simulink model "Quadcopter"  (R2023b)
settings: Solver=VariableStepAuto  StartTime=0.0  StopTime=10  FixedStep=0.002  RelTol=1e-3  EnableMultiTasking=on
libraries: matrix_library x4, shared6dof x1, robotcorelib x1, uavutilslib x1
settings Model: ExtModeTrigDuration=10000  Creator=plad  LastModifiedBy=plad
settings SolverCC: AlgebraicLoopSolver=TrustRegion  PositivePriorityOrder=on
settings DataIOCC: ReturnWorkspaceOutputs=off
settings OptimizationCC: LifeSpan=inf
settings DebuggingCC: UnconnectedInputMsg=warning  UnconnectedOutputMsg=warning  UnconnectedLineMsg=warning  ArithmeticOperatorsInVariantConditions=warning
settings ModelReferenceCC: EnableRefExpFcnMdlSchedulingChecks=on
settings SFSimCC: SimUseLocalCustomCode=off  CustomCodeUndefinedFunction=UseInterfaceOnly
settings RTWCC: Description=QUARC Win64 Target  SystemTargetFile=quarc_win64.tlc  TemplateMakefile=quarc_default_tmf  RTWUseLocalCustomCode=off
settings CodeAppCC: StateflowObjectComments=on
settings STFCustomTargetCC: TargetPreCompLibLocation=C:\PROGRA~3\QUARC\lib\2016a\win64\release  ConcurrentExecutionCompliant=on  GRTInterface=on  SystemTargetFile=quarc_win64.tlc
settings GRTTargetCC: TargetPreCompLibLocation=C:\PROGRA~3\QUARC\lib\2016a\win64\release  ParMdlRefBuildCompliant=off  CompOptLevelCompliant=off  CombineOutputUpdateFcns=off  MatFileLogging=off  CPPClassGenCompliant=off  GRTInterface=on  UseToolchainInfoCompliant=off  ExtMode=on  ExtModeMexFile=quarc_comm
settings ConfigComp: CovMetricSettings=dswe

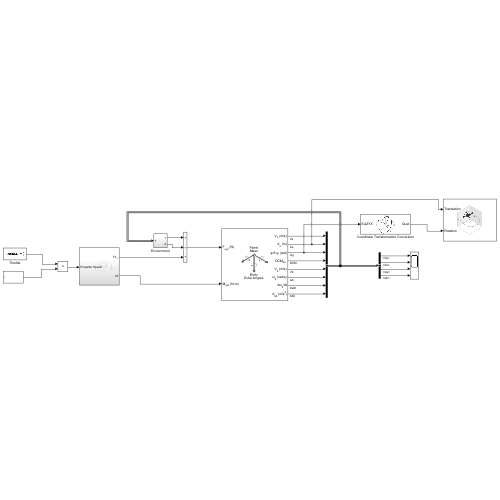
[thumbnail: Simulink's stored preview of the top-level diagram]
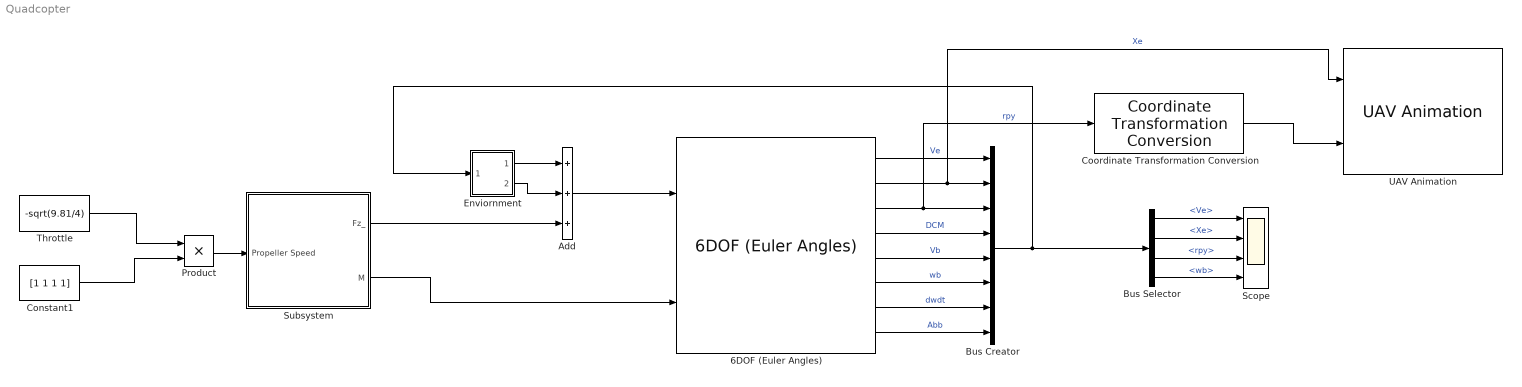
== system Quadcopter ==
  6DOF (Euler Angles) : shared6dof/6DOF (Euler Angles)  units=Metric (MKS)  mtype=Fixed  rep=Euler Angles  xme_0=[0 0 0]  Vm_0=[0 0 0]  eul_0=[0 0 0]  pm_0=[0 0 0]  mass_0=1.0  mass_e=0.5  mass_f=2.0  inertia=eye(3)  inertia_e=eye(3)  inertia_f=2*eye(3)  k_quat=1.0  vre_flag=on  abi_flag=off  aMode=0  xme_statename=''  Vm_statename=''  eul_statename=''  quat_statename=''  pm_statename=''  mass_statename=''
  Add : Sum  Inputs=+++
  Bus Creator : BusCreator  Inputs=8
  Bus Selector : BusSelector  OutputSignals=Ve,Xe,rpy,wb
  Constant1 : Constant  Value=[1 1 1 1]
  Coordinate Transformation Conversion : robotcorelib/Coordinate Transformation Conversion  InputRepresentation=Euler Angles  InputEulerSequence=ZYX  ShowTrVecInputPort=on  OutputRepresentation=Quaternion  OutputEulerSequence=ZYX  ShowTrVecOutputPort=on  SimulateUsing=Interpreted execution
      settings: LibrarySourceBlock=uavutilslib/Coordinate Transformation Conversion
  Enviornment : Subsystem
  Product : Product
  Scope : Scope  NumInputPorts=4
  Subsystem : Subsystem
  Throttle : Constant  Value=-sqrt(9.81/4)
  UAV Animation : uavutilslib/UAV Animation  UAVType=Multirotor  UAVSize=1  InertialZDirection=Down  SampleTime=-1
  wires:
  Bus Selector/1 -> Scope/1  "<Ve>"
  Bus Selector/3 -> Scope/3  "<rpy>"
  Bus Selector/2 -> Scope/2  "<Xe>"
  Bus Creator/1 -> Enviornment/1(In1), Bus Selector/1
  6DOF (Euler Angles)/6 -> Bus Creator/6  "wb"
  6DOF (Euler Angles)/7 -> Bus Creator/7  "dwdt"
  6DOF (Euler Angles)/1 -> Bus Creator/1  "Ve"
  Add/1 -> 6DOF (Euler Angles)/1
  6DOF (Euler Angles)/3 -> Coordinate Transformation Conversion/1, Bus Creator/3  "rpy"
  6DOF (Euler Angles)/4 -> Bus Creator/4  "DCM"
  6DOF (Euler Angles)/5 -> Bus Creator/5  "Vb"
  6DOF (Euler Angles)/8 -> Bus Creator/8  "Abb"
  Throttle/1 -> Product/1
  Bus Selector/4 -> Scope/4  "<wb>"
  6DOF (Euler Angles)/2 -> UAV Animation/1, Bus Creator/2  "Xe"
  Enviornment/1(Out1) -> Add/1
  Enviornment/2(Out2) -> Add/2
  Constant1/1 -> Product/2
  Product/1 -> Subsystem/1(Propeller Speed)
  Subsystem/1(Fz_) -> Add/3
  Subsystem/2(M) -> 6DOF (Euler Angles)/2
  Coordinate Transformation Conversion/1 -> UAV Animation/2

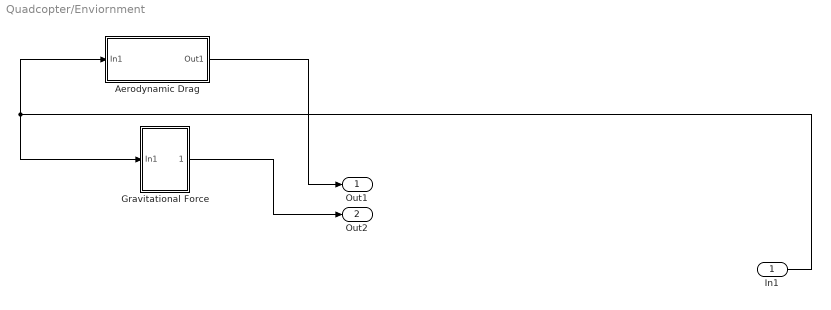
== system Quadcopter/Enviornment ==
  In1 : Inport
  Aerodynamic Drag : Subsystem
  Gravitational Force : Subsystem
  Out1 : Outport
  Out2 : Outport  Port=2
  wires:
  In1/1 -> Aerodynamic Drag/1(In1), Gravitational Force/1(In1)
  Aerodynamic Drag/1(Out1) -> Out1/1
  Gravitational Force/1(Out1) -> Out2/1

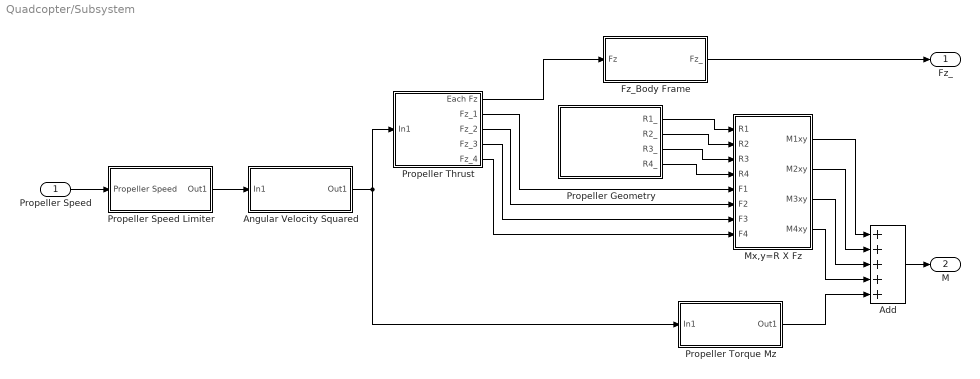
== system Quadcopter/Subsystem ==
  Propeller Speed : Inport
  Add : Sum  Inputs=+++++
  Angular Velocity Squared : Subsystem
  Fz_Body Frame : Subsystem
  Mx,y=R X Fz : Subsystem
  Propeller Geometry : Subsystem
  Propeller Speed Limiter : Subsystem
  Propeller Thrust : Subsystem
  Propeller Torque Mz : Subsystem
  Fz_ : Outport
  M : Outport  Port=2
  wires:
  Propeller Speed/1 -> Propeller Speed Limiter/1(Propeller Speed)
  Propeller Speed Limiter/1(Out1) -> Angular Velocity Squared/1(In1)
  Angular Velocity Squared/1(Out1) -> Propeller Torque Mz/1(In1), Propeller Thrust/1(In1)
  Add/1 -> M/1
  Propeller Torque Mz/1(Out1) -> Add/5
  Propeller Geometry/1(R1_) -> Mx,y=R X Fz/1(R1)
  Propeller Geometry/2(R2_) -> Mx,y=R X Fz/2(R2)
  Propeller Geometry/3(R3_) -> Mx,y=R X Fz/3(R3)
  Propeller Geometry/4(R4_) -> Mx,y=R X Fz/4(R4)
  Propeller Thrust/1(Each Fz) -> Fz_Body Frame/1(Fz)
  Propeller Thrust/2(Fz_1) -> Mx,y=R X Fz/5(F1)
  Propeller Thrust/3(Fz_2) -> Mx,y=R X Fz/6(F2)
  Propeller Thrust/4(Fz_3) -> Mx,y=R X Fz/7(F3)
  Propeller Thrust/5(Fz_4) -> Mx,y=R X Fz/8(F4)
  Fz_Body Frame/1(Fz_) -> Fz_/1
  Mx,y=R X Fz/1(M1xy) -> Add/1
  Mx,y=R X Fz/2(M2xy) -> Add/2
  Mx,y=R X Fz/3(M3xy) -> Add/3
  Mx,y=R X Fz/4(M4xy) -> Add/4

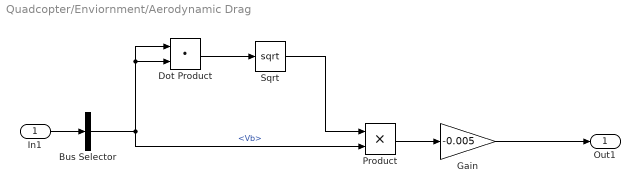
== system Quadcopter/Enviornment/Aerodynamic Drag ==
  In1 : Inport
  Bus Selector : BusSelector  OutputSignals=Vb
  Dot Product : DotProduct  OutDataTypeStr=Inherit: Inherit via internal rule
  Gain : Gain  Gain=-0.005
  Product : Product
  Sqrt : Sqrt
  Out1 : Outport
  wires:
  In1/1 -> Bus Selector/1
  Bus Selector/1 -> Dot Product/1, Dot Product/2, Product/2  "<Vb>"
  Dot Product/1 -> Sqrt/1
  Sqrt/1 -> Product/1
  Product/1 -> Gain/1
  Gain/1 -> Out1/1

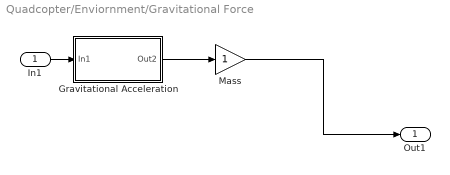
== system Quadcopter/Enviornment/Gravitational Force ==
  In1 : Inport
  Gravitational Acceleration : Subsystem
  Mass : Gain
  Out1 : Outport
  wires:
  In1/1 -> Gravitational Acceleration/1(In1)
  Gravitational Acceleration/1(Out2) -> Mass/1
  Mass/1 -> Out1/1

== system Quadcopter/Subsystem/Angular Velocity Squared ==
  In1 : Inport
  Abs : Abs  SaturateOnIntegerOverflow=off
  Product : Product
  Out1 : Outport
  wires:
  Abs/1 -> Product/1
  Product/1 -> Out1/1
  In1/1 -> Product/2, Abs/1

== system Quadcopter/Subsystem/Fz_Body Frame ==
  Fz : Inport
  Sum of Elements : Sum  Inputs=+
  z-vector : Subsystem
  Fz_ : Outport
  wires:
  Fz/1 -> Sum of Elements/1
  z-vector/1(Fz_out) -> Fz_/1
  Sum of Elements/1 -> z-vector/1(Fz_in)

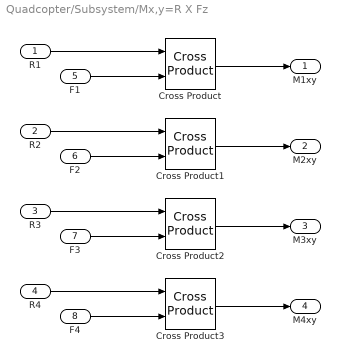
== system Quadcopter/Subsystem/Mx,y=R X Fz ==
  R1 : Inport
  R2 : Inport  Port=2
  R3 : Inport  Port=3
  R4 : Inport  Port=4
  F1 : Inport  Port=5
  F2 : Inport  Port=6
  F3 : Inport  Port=7
  F4 : Inport  Port=8
  Cross Product{,1..3} (4 alike) : matrix_library/Cross Product
  M1xy : Outport
  M2xy : Outport  Port=2
  M3xy : Outport  Port=3
  M4xy : Outport  Port=4
  wires:
  R1/1 -> Cross Product/1
  F1/1 -> Cross Product/2
  R2/1 -> Cross Product1/1
  F2/1 -> Cross Product1/2
  R3/1 -> Cross Product2/1
  F3/1 -> Cross Product2/2
  R4/1 -> Cross Product3/1
  F4/1 -> Cross Product3/2
  Cross Product/1 -> M1xy/1
  Cross Product1/1 -> M2xy/1
  Cross Product2/1 -> M3xy/1
  Cross Product3/1 -> M4xy/1

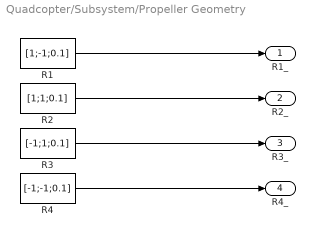
== system Quadcopter/Subsystem/Propeller Geometry ==
  R1 : Constant  Value=[1;-1;0.1]
  R2 : Constant  Value=[1;1;0.1]
  R3 : Constant  Value=[-1;1;0.1]
  R4 : Constant  Value=[-1;-1;0.1]
  R1_ : Outport
  R2_ : Outport  Port=2
  R3_ : Outport  Port=3
  R4_ : Outport  Port=4
  wires:
  R1/1 -> R1_/1
  R2/1 -> R2_/1
  R3/1 -> R3_/1
  R4/1 -> R4_/1

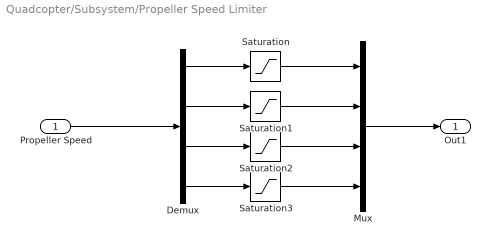
== system Quadcopter/Subsystem/Propeller Speed Limiter ==
  Propeller Speed : Inport
  Demux : Demux
  Mux : Mux
  Saturation{,1..3} (4 alike) : Saturate  UpperLimit=300  LowerLimit=-300
  Out1 : Outport
  wires:
  Propeller Speed/1 -> Demux/1
  Demux/1 -> Saturation/1
  Saturation/1 -> Mux/1
  Demux/2 -> Saturation1/1
  Demux/3 -> Saturation2/1
  Demux/4 -> Saturation3/1
  Saturation1/1 -> Mux/2
  Saturation2/1 -> Mux/3
  Saturation3/1 -> Mux/4
  Mux/1 -> Out1/1

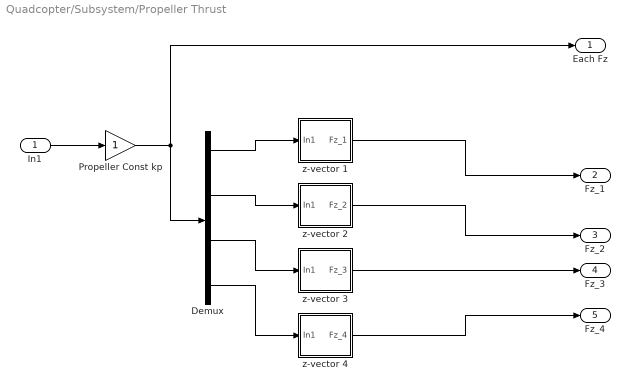
== system Quadcopter/Subsystem/Propeller Thrust ==
  In1 : Inport
  Demux : Demux
  Propeller Const kp : Gain
  z-vector 1 : Subsystem
  z-vector 2 : Subsystem
  z-vector 3 : Subsystem
  z-vector 4 : Subsystem
  Each Fz : Outport
  Fz_1 : Outport  Port=2
  Fz_2 : Outport  Port=3
  Fz_3 : Outport  Port=4
  Fz_4 : Outport  Port=5
  wires:
  In1/1 -> Propeller Const kp/1
  Propeller Const kp/1 -> Demux/1, Each Fz/1
  Demux/1 -> z-vector 1/1(In1)
  Demux/2 -> z-vector 2/1(In1)
  Demux/3 -> z-vector 3/1(In1)
  Demux/4 -> z-vector 4/1(In1)
  z-vector 1/1(Fz_1) -> Fz_1/1
  z-vector 2/1(Fz_2) -> Fz_2/1
  z-vector 3/1(Fz_3) -> Fz_3/1
  z-vector 4/1(Fz_4) -> Fz_4/1

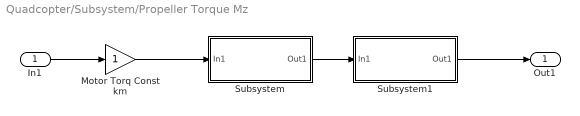
== system Quadcopter/Subsystem/Propeller Torque Mz ==
  In1 : Inport
  Motor Torq Const km : Gain
  Subsystem : Subsystem
  Subsystem1 : Subsystem
  Out1 : Outport
  wires:
  In1/1 -> Motor Torq Const km/1
  Motor Torq Const km/1 -> Subsystem/1(In1)
  Subsystem/1(Out1) -> Subsystem1/1(In1)
  Subsystem1/1(Out1) -> Out1/1

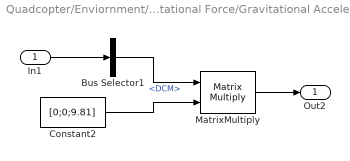
== system Quadcopter/Enviornment/Gravitational Force/Gravitational Acceleration ==
  In1 : Inport
  Bus Selector1 : BusSelector  OutputSignals=DCM
  Constant2 : Constant  Value=[0;0;9.81]
  MatrixMultiply : Product  Multiplication=Matrix(*)
  Out2 : Outport
  wires:
  In1/1 -> Bus Selector1/1
  Bus Selector1/1 -> MatrixMultiply/1  "<DCM>"
  Constant2/1 -> MatrixMultiply/2
  MatrixMultiply/1 -> Out2/1

== system Quadcopter/Subsystem/Fz_Body Frame/z-vector ==
  Fz_in : Inport
  Constant : Constant  Value=[0;0;1]
  Product : Product
  Fz_out : Outport
  wires:
  Constant/1 -> Product/1
  Fz_in/1 -> Product/2
  Product/1 -> Fz_out/1

== system Quadcopter/Subsystem/Propeller Thrust/z-vector 1 ==
  In1 : Inport
  Product : Product
  az : Constant  Value=[0;0;1]
  Fz_1 : Outport
  wires:
  az/1 -> Product/1
  In1/1 -> Product/2
  Product/1 -> Fz_1/1

== system Quadcopter/Subsystem/Propeller Thrust/z-vector 2 ==
  In1 : Inport
  Product : Product
  az : Constant  Value=[0;0;1]
  Fz_2 : Outport
  wires:
  Product/1 -> Fz_2/1
  In1/1 -> Product/2
  az/1 -> Product/1

== system Quadcopter/Subsystem/Propeller Thrust/z-vector 3 ==
  In1 : Inport
  Product : Product
  az : Constant  Value=[0;0;1]
  Fz_3 : Outport
  wires:
  az/1 -> Product/1
  In1/1 -> Product/2
  Product/1 -> Fz_3/1

== system Quadcopter/Subsystem/Propeller Thrust/z-vector 4 ==
  In1 : Inport
  Product : Product
  az : Constant  Value=[0;0;1]
  Fz_4 : Outport
  wires:
  Product/1 -> Fz_4/1
  In1/1 -> Product/2
  az/1 -> Product/1

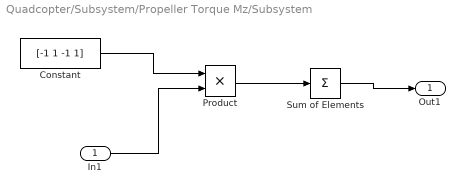
== system Quadcopter/Subsystem/Propeller Torque Mz/Subsystem ==
  In1 : Inport
  Constant : Constant  Value=[-1 1 -1 1]
  Product : Product
  Sum of Elements : Sum  Inputs=+
  Out1 : Outport
  wires:
  Constant/1 -> Product/1
  In1/1 -> Product/2
  Product/1 -> Sum of Elements/1
  Sum of Elements/1 -> Out1/1

== system Quadcopter/Subsystem/Propeller Torque Mz/Subsystem1 ==
  In1 : Inport
  Constant : Constant  Value=[0;0;1]
  Product : Product
  Out1 : Outport
  wires:
  Constant/1 -> Product/1
  In1/1 -> Product/2
  Product/1 -> Out1/1
